simulink model "rlClheroRobot"  (R2020a)
settings: Solver=VariableStepAuto  StartTime=0.0  StopTime=10.0  RelTol=1e-3
values from neighbouring files (symbols this model uses):
  dist1 = 275    [Parametros_RHex.m]
  espesor = 10    [Parametros_RHex.m]
  init_height = h    (= 4)    [Parametros_RHex.m]
  masa_C_Leg = 0.057    [Parametros_RHex.m]
  radio = 100    [Parametros_RHex.m]
  Tf = 10    [Parametros_RHex.m]
  Ts = 0.025    [Parametros_RHex.m]
undefined symbols (not defined in the file or in its folder): X, Y, Z
libraries: nesl_utility x44, sm_lib x35, Contact_Forces_Lib x22, simulink x7, rllib x1
(part 3 of 3)

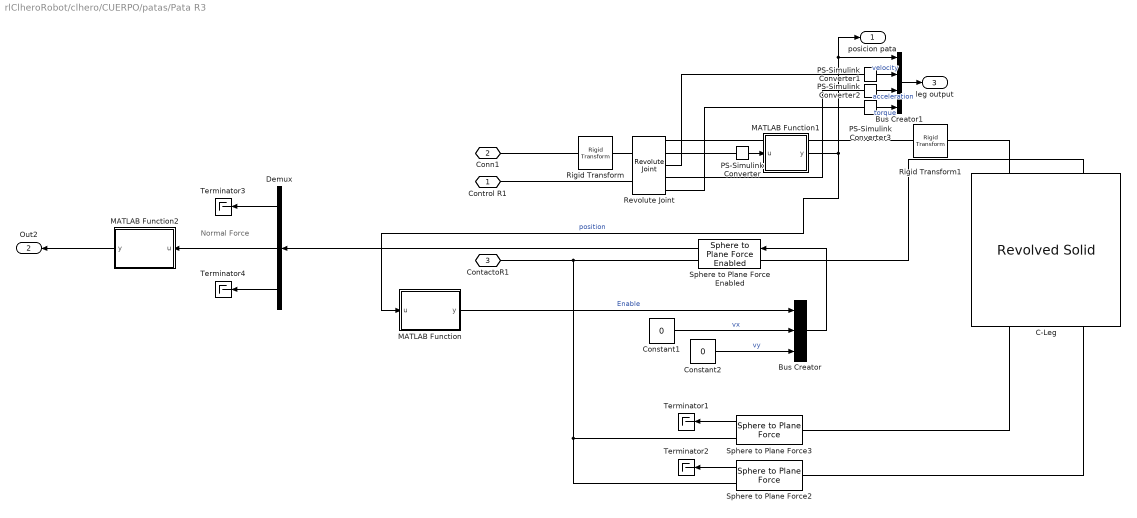
== system rlClheroRobot/clhero/CUERPO/patas/Pata R3 ==
  note: Normal Force
  Bus Creator : BusCreator  Inputs=3
  Bus Creator1 : BusCreator  Inputs=4
  C-Leg : sm_lib/Body Elements/Revolved Solid  GraphicAmbientColor=[0.15 0.15 0.15 1.0]  BasedOnType=Mass  CenterOfMass=[-42.439/1000 25/1000 -108.743/1000]  CenterOfMassUnits=mm  GraphicDiffuseColor=[1.0 0.2 0.0]  ExportConvexHullGeometry=off  Density=1000  DensityUnits=kg/m^3  DoExposeReferenceFrame=on  GraphicEmissiveColor=[0.0 0.0 0.0 1.0]  ExportEntireGeometry=off  SerializedFrames=<Frames><Frame><Id>Frame1</Id><Value><Name>F1</Name><Origin><Source>GeometricFeature</Source><FeatureName>front point 2</FeatureName></Origin><PrimaryAxis><DefinedDirection>+Z</DefinedDirection><Source>ReferenceFrame</Source><SourceDirection>+Z</SourceDirection><FeatureName></FeatureName></PrimaryAxis><SecondaryAxis><DefinedDirection>+X</DefinedDirection><Source>ReferenceFrame</Source><SourceDirection>+X</SourceDirection><FeatureName></FeatureName></SecondaryAxis></Value></Frame><Frame><Id>Frame2</Id><Value><Name>F2</Name><Origin><Source>GeometricFeature</Source><FeatureName>front point 3</FeatureName></Origin><PrimaryAxis><DefinedDirection>+Z</DefinedDirection><Source>ReferenceFrame</Source><SourceDirection>+Z</SourceDirection><FeatureName></FeatureName></PrimaryAxis><SecondaryAxis><DefinedDirection>+X</DefinedDirection><Source>ReferenceFrame</Source><SourceDirection>+X</SourceDirection><FeatureName></FeatureName></SecondaryAxis></Value></Frame><Frame><Id>Frame3</Id><Value><Name>F3</Name><Origin><Source>GeometricFeature</Source><FeatureName>side surface 2</FeatureName></Origin><PrimaryAxis><DefinedDirection>+Z</DefinedDirection><Source>ReferenceFrame</Source><SourceDirection>+Z</SourceDirection><FeatureName></FeatureName></PrimaryAxis><SecondaryAxis><DefinedDirection>+X</DefinedDirection><Source>ReferenceFrame</Source><SourceDirection>+X</SourceDirection><FeatureName></FeatureName></SecondaryAxis></Value></Frame></Frames>  MarkerShape=Sphere  MarkerSize=10  GraphicType=FromGeometry  InertiaType=Custom  Mass=masa_C_Leg  MassUnits=kg  MomentsOfInertia=[0.001038176 0.000273753 0.001217746]  MomentsOfInertiaUnits=kg*mm^2  GraphicOpacity=1.0  ProductsOfInertia=[-0.000218169 0.000059956 0.000153627]  ProductsOfInertiaUnits=kg*mm^2  RevolutionCrossSection=perfil_C_Leg  RevolutionCrossSectionUnits=mm  RevolutionAngle=240  RevolutionAngleUnits=deg  RevolutionExtent=Custom  GraphicShininess=75  GraphicSpecularColor=[0.5 0.5 0.5 1.0]  GraphicVisPropType=SimpleVisualProperties
  Constant1 : Constant  Value=0
  Constant2 : Constant  Value=0
  Demux : Demux  Outputs=3
  MATLAB Function : MATLAB Function  TreatAsAtomicUnit=on
  MATLAB Function1 : MATLAB Function  TreatAsAtomicUnit=on
  MATLAB Function2 : MATLAB Function  TreatAsAtomicUnit=on
  PS-Simulink Converter : nesl_utility/PS-Simulink Converter  PhysicalDomain=network_engine_domain  SubClassName=ps_output  LeftPortType=input  RightPortType=output  PseudoPeriodic=off  Frequencies=[]  Unit=rad  AffineConversion=off
  PS-Simulink Converter1 : nesl_utility/PS-Simulink Converter  PhysicalDomain=network_engine_domain  SubClassName=ps_output  LeftPortType=input  RightPortType=output  PseudoPeriodic=off  Frequencies=[]  Unit=rad/s  AffineConversion=off
  PS-Simulink Converter2 : nesl_utility/PS-Simulink Converter  PhysicalDomain=network_engine_domain  SubClassName=ps_output  LeftPortType=input  RightPortType=output  PseudoPeriodic=off  Frequencies=[]  Unit=1  AffineConversion=off
  PS-Simulink Converter3 : nesl_utility/PS-Simulink Converter  PhysicalDomain=network_engine_domain  SubClassName=ps_output  LeftPortType=input  RightPortType=output  PseudoPeriodic=off  Frequencies=[]  Unit=N*m  AffineConversion=off
  Revolute Joint : sm_lib/Joints/Revolute Joint  JointMode=Normal  SenseConstraintForce=off  SenseConstraintForceX=off  SenseConstraintForceY=off  SenseConstraintForceZ=off  SenseConstraintTorque=off  SenseConstraintTorqueX=off  SenseConstraintTorqueY=off  SenseConstraintTorqueZ=off  SenseTotalForce=off  SenseTotalForceX=off  SenseTotalForceY=off  SenseTotalForceZ=off  SenseTotalTorque=off  SenseTotalTorqueX=off  SenseTotalTorqueY=off  SenseTotalTorqueZ=off  CompositeWrenchDir=FollowerOnBase  CompositeWrenchFrame=BaseFrame  EquilibriumPosition=0  EquilibriumPositionUnits=deg  SpringStiffness=0  SpringStiffnessUnits=N*m/deg  DampingCoefficient=0  DampingCoefficientUnits=N*m/(deg/s)  TorqueActuationMode=ComputedTorque  MotionActuationMode=InputMotion  SensePosition=on  SenseVelocity=on  SenseAcceleration=on  SenseTorqueForce=on  SenseLowerLimitTorqueForce=off  SenseUpperLimitTorqueForce=off  LowerLimitSpecify=off  LowerLimitBound=-90  LowerLimitBoundUnits=deg  LowerLimitStiffness=1e4  LowerLimitStiffnessUnits=N*m/deg  LowerLimitDamping=10  LowerLimitDampingUnits=N*m/(deg/s)  LowerLimitTransitionRegionWidth=0.1  LowerLimitTransitionRegionWidthUnits=deg  UpperLimitSpecify=off  UpperLimitBound=90  UpperLimitBoundUnits=deg  UpperLimitStiffness=1e4  UpperLimitStiffnessUnits=N*m/deg  UpperLimitDamping=10  UpperLimitDampingUnits=N*m/(deg/s)  UpperLimitTransitionRegionWidth=0.1  UpperLimitTransitionRegionWidthUnits=deg  PositionTargetSpecify=on  PositionTargetPriority=High  PositionTargetValue=leg_initial_pose  PositionTargetValueUnits=rad  VelocityTargetSpecify=off  VelocityTargetPriority=High  VelocityTargetValue=0  VelocityTargetValueUnits=deg/s
  Rigid Transform : sm_lib/Frames and Transforms/Rigid Transform  TranslationMethod=Cartesian  TranslationStandardOffset=0  TranslationLengthUnit=cm  TranslationStandardAxis=+Y  TranslationCartesianOffset=[23.635 27.496 0]  TranslationROffset=0  TranslationROffsetUnits=m  TranslationZOffset=0  TranslationZOffsetUnits=m  TranslationThetaOffset=0  TranslationThetaOffsetUnits=deg  RotationMethod=StandardAxis  RotationAngleUnits=deg  RotationStandardAxis=+X  RotationAngle=90  RotationArbitraryAxis=[0 0 1]  FollAlignAxisA=-Z  BaseAlignAxisA=+X  FollAlignAxisB=+X  BaseAlignAxisB=+Z  RotationSequenceAxes=FollowerAxes  RotationSequence=XYX  RotationSequenceAngles=[0 0 0]  RotationSequenceAnglesUnits=deg  RotationMatrix=[1 0 0; 0 1 0; 0 0 1]
  Rigid Transform1 : sm_lib/Frames and Transforms/Rigid Transform  TranslationMethod=Cylindrical  TranslationStandardOffset=0  TranslationLengthUnit=mm  TranslationStandardAxis=+Z  TranslationCartesianOffset=[0 -(dist1/2)-radio+(espesor/2) 0]  TranslationROffset=radio-espesor/2  TranslationROffsetUnits=mm  TranslationZOffset=0  TranslationZOffsetUnits=m  TranslationThetaOffset=-120  TranslationThetaOffsetUnits=deg  RotationMethod=StandardAxis  RotationAngleUnits=rad  RotationStandardAxis=+Z  RotationAngle=0  RotationArbitraryAxis=[0 0 1]  FollAlignAxisA=-Z  BaseAlignAxisA=+X  FollAlignAxisB=+X  BaseAlignAxisB=+Z  RotationSequenceAxes=FollowerAxes  RotationSequence=XYX  RotationSequenceAngles=[0 0 0]  RotationSequenceAnglesUnits=deg  RotationMatrix=[1 0 0; 0 1 0; 0 0 1]
  Sphere to Plane Force Enabled : Contact_Forces_Lib/3D/Sphere to Plane Force Enabled  sphere_rad=radio/1000  plane_lenx=10  plane_leny=10  plane_depth=0.05/2  force_law=Linear  k_contact=cont1  b_contact=cont2  pen_full_damp_F=0  pen_exponent=1  custom_param_1=1  custom_param_2=1  friction_law=Stick-Slip Continuous  mu_kinetic=fric1  mu_static=fric2  v_thr=0.1  vis_on=off  vis_opc_en=0  vis_len_plaBz=0.005  vis_clr=[0.9 0.2 0.2]  vis_opc=0.7
      settings: SourceProductName=Simscape Multibody Contact Forces Library
  Sphere to Plane Force2 : Contact_Forces_Lib/3D/Sphere to Plane Force  sphere_rad=1e-6  plane_lenx=10  plane_leny=10  plane_depth=0.025  force_law=Linear  k_contact=cont1  b_contact=cont2  pen_full_damp_F=1e-4  pen_exponent=1  custom_param_1=1  custom_param_2=1  friction_law=Stick-Slip Continuous  mu_kinetic=fric1  mu_static=fric2  v_thr=0.1  vis_on=off  vis_opc_en=0  vis_len_plaBz=0.005  vis_clr=[0.9 0.2 0.2]  vis_opc=0.7
  Sphere to Plane Force3 : Contact_Forces_Lib/3D/Sphere to Plane Force  sphere_rad=1e-6  plane_lenx=10  plane_leny=10  plane_depth=0.025  force_law=Linear  k_contact=cont1  b_contact=cont2  pen_full_damp_F=1e-4  pen_exponent=1  custom_param_1=1  custom_param_2=1  friction_law=Stick-Slip Continuous  mu_kinetic=fric1  mu_static=fric2  v_thr=0.1  vis_on=off  vis_opc_en=0  vis_len_plaBz=0.005  vis_clr=[0.9 0.2 0.2]  vis_opc=0.7
  Terminator{1..4} (4 alike) : Terminator
  Control R1 : PMIOPort  Side=Right
  Conn1 : PMIOPort  Port=2  Side=Left
  ContactoR1 : PMIOPort  Port=3  Side=Right
  posicion pata : Outport  VectorParamsAs1DForOutWhenUnconnected=off
  Out2 : Outport  Port=2  VectorParamsAs1DForOutWhenUnconnected=off
  leg output : Outport  Port=3
  wires:
  Constant1/1 -> Bus Creator/2  "vx"
  Constant2/1 -> Bus Creator/3  "vy"
  MATLAB Function/1(y) -> Bus Creator/1  "Enable"
  PS-Simulink Converter/1 -> MATLAB Function1/1(u)
  MATLAB Function1/1(y) -> MATLAB Function/1(u), Bus Creator1/1, posicion pata/1  "position"
  Sphere to Plane Force2/1 -> Terminator2/1
  Sphere to Plane Force3/1 -> Terminator1/1
  Bus Creator/1 -> Sphere to Plane Force Enabled/1
  Sphere to Plane Force Enabled/1 -> Demux/1
  Demux/1 -> Terminator3/1
  Demux/2 -> MATLAB Function2/1(u)
  Demux/3 -> Terminator4/1
  MATLAB Function2/1(y) -> Out2/1
  Bus Creator1/1 -> leg output/1
  PS-Simulink Converter1/1 -> Bus Creator1/2  "velocity"
  PS-Simulink Converter2/1 -> Bus Creator1/3  "acceleration"
  PS-Simulink Converter3/1 -> Bus Creator1/4  "torque"
  connections:
  Revolute Joint/LConn1 -- Rigid Transform/RConn1
  Rigid Transform1/RConn1 -- Revolute Joint/RConn1
  Rigid Transform/LConn1 -- Conn1/RConn1
  Revolute Joint/LConn2 -- Control R1/RConn1
  Sphere to Plane Force3/RConn1 -- Sphere to Plane Force2/RConn1 -- Sphere to Plane Force Enabled/RConn1 -- ContactoR1/RConn1
  Revolute Joint/RConn2 -- PS-Simulink Converter/LConn1
  C-Leg/LConn1 -- Sphere to Plane Force3/LConn1
  Sphere to Plane Force2/LConn1 -- C-Leg/LConn2
  C-Leg/RConn1 -- Rigid Transform1/LConn1
  Sphere to Plane Force Enabled/LConn1 -- C-Leg/RConn2
  Revolute Joint/RConn3 -- PS-Simulink Converter1/LConn1
  PS-Simulink Converter2/LConn1 -- Revolute Joint/RConn4
  Revolute Joint/RConn5 -- PS-Simulink Converter3/LConn1

== matlab function rlClheroRobot/clhero/CUERPO/patas/Pata L2/MATLAB Function2 ==
  data: u input; y output
function y = fcn(u)
if u~=0
    y=1;
else
    y=0;

end

== matlab function rlClheroRobot/clhero/CUERPO/patas/Pata R2/MATLAB Function2 ==
  data: u input; y output
function y = fcn(u)
if u~=0
    y=1;
else
    y=0;

end

== matlab function rlClheroRobot/clhero/CUERPO/patas/Pata R1/MATLAB Function2 ==
  data: u input; y output
function y = fcn(u)
if u~=0
    y=1;
else
    y=0;

end

== matlab function rlClheroRobot/clhero/CUERPO/patas/Pata R3/MATLAB Function2 ==
  data: u input; y output
function y = fcn(u)
if u~=0
    y=1;
else
    y=0;

end

== matlab function rlClheroRobot/clhero/CUERPO/Rotation Matrix to Yaw Pitch Roll ==
  data: q input; eul output
function eul = calcAttitude(q)

% Normalize the quaternions
q = bsxfun(@times, q, 1./sqrt(sum(q.^2,1)));
qw = q(1);
qx = q(2);
qy = q(3);
qz = q(4);

% Pre-allocate output
eul = zeros(3, 1, 'like', q);

aSinInput = -2*(qx.*qz-qw.*qy);
aSinInput(aSinInput > 1) = 1;
aSinInput(aSinInput < -1) = -1;

eul = [ atan2( 2*(qx.*qy+qw.*qz), qw.^2 + qx.^2 - qy.^2 - qz.^2 ); ...
    asin( aSinInput ); ...
    atan2( 2*(qy.*qz+qw.*qx), qw.^2 - qx.^2 - qy.^2 + qz.^2 )];

== matlab function rlClheroRobot/clhero/CUERPO/patas/Pata L1/MATLAB Function ==
  data: u input; y output
function y = fcn(u)
int8 y
if u>1.43 && u<2.683

    y=0;
else
    y=1;

end

== matlab function rlClheroRobot/clhero/CUERPO/patas/Pata L3/MATLAB Function ==
  data: u input; y output
function y = fcn(u)
int8 y
if u>1.43 && u<2.683

    y=0;
else
    y=1;

end

== matlab function rlClheroRobot/clhero/CUERPO/patas/Pata L3/MATLAB Function1 ==
  data: u input; y output
function y = fcn(u)

y = mod(u,2*pi);

== matlab function rlClheroRobot/clhero/CUERPO/patas/Pata L2/MATLAB Function ==
  data: u input; y output
function y = fcn(u)
int8 y
if u>1.43 && u<2.683

    y=0;
else
    y=1;

end

== matlab function rlClheroRobot/clhero/CUERPO/patas/Pata L2/MATLAB Function1 ==
  data: u input; y output
function y = fcn(u)

y = mod(u,2*pi);

== matlab function rlClheroRobot/clhero/CUERPO/patas/Pata R2/MATLAB Function ==
  data: u input; y output
function y = fcn(u)
int8 y
if u>1.43 && u<2.683

    y=0;
else
    y=1;

end

== matlab function rlClheroRobot/clhero/CUERPO/patas/Pata R2/MATLAB Function1 ==
  data: u input; y output
function y = fcn(u)

y = mod(u,2*pi);

== matlab function rlClheroRobot/clhero/CUERPO/patas/Pata R1/MATLAB Function ==
  data: u input; y output
function y = fcn(u)
int8 y
if u>1.43 && u<2.683

    y=0;
else
    y=1;

end

== matlab function rlClheroRobot/clhero/CUERPO/patas/Pata L1/MATLAB Function1 ==
  data: u input; y output
function y = fcn(u)

y = mod(u,2*pi);

== matlab function rlClheroRobot/clhero/CUERPO/patas/Pata R1/MATLAB Function1 ==
  data: u input; y output
function y = fcn(u)

y = mod(u,2*pi);

== matlab function rlClheroRobot/clhero/CUERPO/patas/Pata R3/MATLAB Function ==
  data: u input; y output
function y = fcn(u)
int8 y
if u>1.43 && u<2.683

    y=0;
else
    y=1;

end

== matlab function rlClheroRobot/clhero/CUERPO/patas/Pata R3/MATLAB Function1 ==
  data: u input; y output
function y = fcn(u)

y = mod(u,2*pi);

== matlab function rlClheroRobot/clhero/CUERPO/patas/Pata L1/MATLAB Function2 ==
  data: u input; y output
function y = fcn(u)
if u~=0
    y=1;
else
    y=0;

end

== matlab function rlClheroRobot/clhero/CUERPO/patas/Pata L3/MATLAB Function2 ==
  data: u input; y output
function y = fcn(u)
if u~=0
    y=1;
else
    y=0;

end
